simulink model "RL_Traction_motor_torch"  (R2022a)
settings: Solver=FixedStepAuto  StartTime=0.0  StopTime=0.25  FixedStep=5E-6  RelTol=1e-3
model workspace (MAT data in the model file):
  Cdc = 0.001
  Jm = 0.1234
  Ki_id = 710.3004
  Ki_iq = 1061.5
  Ki_omega = 500
  Kp_id = 0.8779
  Kp_iq = 1.0744
  Kp_omega = 20
  L0 = 0.00012184
  Ld = 0.00024368
  LdMatrix = [0.000182 0.00018 0.000178 0.000177 0.000176 0.00017475 0.0001735 0.00017247 0.00017132 0.00016571 0.00016537 0.00016571 ... (735 elements, 21x35)]
  Lq = 0.00029758
  LqMatrix = [0.000217 0.000217 0.000217 0.000217 0.000217 0.0002145 0.000212 0.0002115 0.00021022 0.0002079 0.00020461 0.0002079 ... (735 elements, 21x35)]
  PmMatrix = [0.0363 0.0363 0.0363 0.0363 0.0363 0.0363 0.0363 0.0363 0.0363 0.0363 0.0363 0.0363 ... (735 elements, 21x35)]
  Pmax = 35000
  Rs = 0.010087
  Tmax = 200
  Ts = 5e-06
  Tsc = 0.0001
  V1 = 290
  Vnom = 325
  fsw = 10000
  idVec = [-250 -225 -200 -175 -150 -125 -100 -75 -50 -25 0 25 50 75 100 125 150 175 200 225 250]
  iqVec = [-425 -400 -375 -350 -325 -300 -275 -250 -225 -200 -175 -150 -125 -100 -75 -50 -25 0 25 50 75 100 125 150 175 200 225 250 275 300 325 350 375 400 425]
  p = 8
  psim = 0.044
undefined symbols (not defined in the file or in its folder): ee_sli_rtmsupport, gcbh, idMatrix, Imax, iqMatrix, rpmVec, TqVec, VdcVec
libraries: fl_lib x19, nesl_utility x13, eeGeneralControl x9, ee_lib x7, slpidlib x5, simulink x3, eeTransforms x2, eeDqVoltageLimiter x1, eePwmGeneratorTwoLevel x1, eeResolverToDigitalConverter x1
(part 1 of 3)
settings Model: Creator=USER  LastModifiedBy=USER
settings DataIOCC: ReturnWorkspaceOutputs=off
settings ModelReferenceCC: EnableRefExpFcnMdlSchedulingChecks=off
settings RTWCC: Description=Generic Real-Time Target

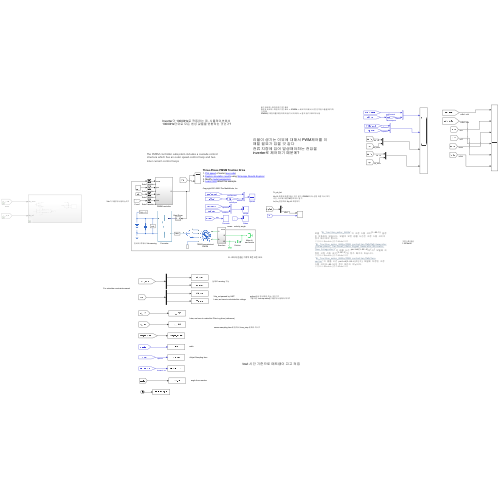
[thumbnail: Simulink's stored preview of the top-level diagram]
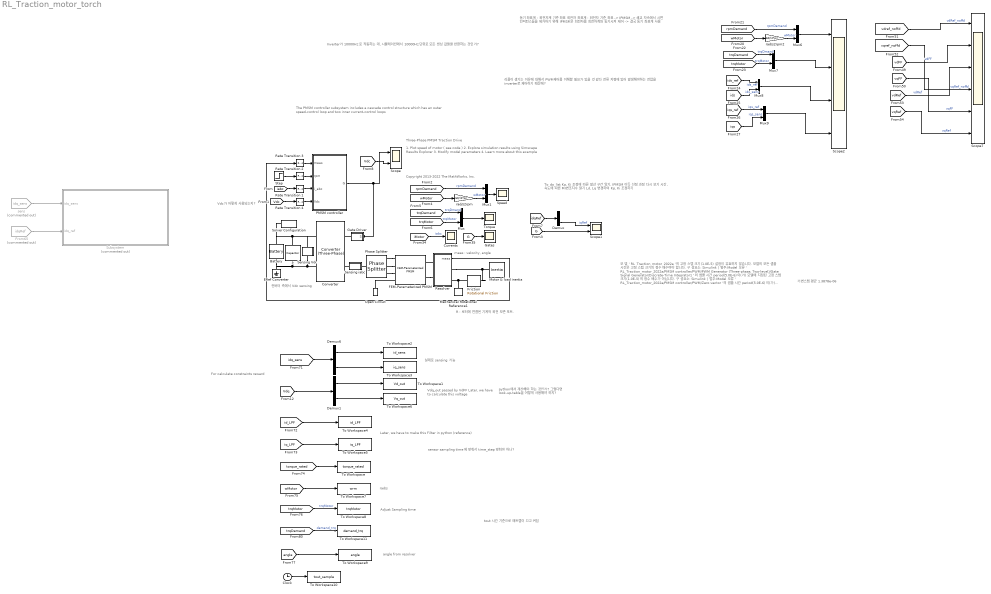
== system RL_Traction_motor_torch ==
  note: 가변스텝 평균
      | 1.3878e-06
  note: 모 델 ' RL_Traction_motor_2022a '의 고정 스텝 크기(1.0E-5) 설정이 유효하지 않습니다. 모델의 모든 샘플 시간은 고정 스텝 크기의 정수 배수여야 합니다.
      | 구 성요소: Simulink | 범주:Model 오류
      | ' RL_Traction_motor_2022a/PMSM controller/PWM/PWM Generator (Three-phase, Two-level)/Gate Signal Generator/Discrete-Time Integrator1 '의 샘플 시간 period(5.0E-6)이(가) 모델에 지정된 고정 스텝 크기(1.0E-5)의 정수 배수가 아닙니다.
      | 구 성요소: Simulink | 범주:Model 오류
      | ' RL_Traction_motor_2022a/PMSM controller/PWM/Zero vector '의 샘플 시간 period(5.0E-6)이(가) 모델에 지정된 고정 스텝 크기(1.0E-5)의 정수 배수가 아닙니다.
      | 구 성요소: Simulink | 범주:Model 오류
  note: Later, we have to make this Filter in python (reference)
  note: python에서 계산해야 하는 것인가?
      | 그렇다면 look-up-table을 어떻게 사용해야 하지?
  note: tout 시간 기준으로 매트랩이 끄고 켜짐
  note: sensor sampling time에 맞춰서 time_step 맞춰야 하나?
  note: 동기 좌표계 : 회전자계 기준 좌표
      | 회전자 좌표계 : 회전자 기준 좌표 -> IPMSM -> 쇄교 자속에서 시변 인덕턴스들을 제거하기 위해
      | IPMSM은 회전자를 회전자계와 동기시켜 제어 -> 결국 동기 좌표계 사용
  note: angle from resolver
  note: rad/s
  note: Adjust Sampling time
  note: 실제로 sensing 가능
  note: For calculate constraints reward
  note: Vdq_out passed by VdFF
      | Later, we have to calculate this voltage
  note: Inverter가 10000Hz로 작동하는 데, 시뮬레이션에서 10000Hz단위로 모든 센싱 값들을 반환하는 것인가?
  note: 리플이 생기는 이유에 대해서 PWM제어를 이해할 필요가 있을 것 같다
      | 전류 지령에 있어 발생해야하는 전압을 inverter로 제어하기 때문에?
  note: To_do_list
      |
      | Kp, Ki 조정에 따른 발산 구간 알기, IPMSM 이득 선정 과정 다시 보기
      | 시간, 속도에 따른 MI변조지수 알기
      | Ld, Lq 변경하여 Kp, Ki 조정하기
  note: Vdc가 어떻게 사용되는지?
  note: R : 로터에 연결된 기계적 회전 보존 포트.
  note: 컨버터 측에서 Vdc sensing
  note: The PMSM controller subsystem includes a cascade control structure which has an outer speed-control loop and two inner current-control loops
  note: Copyright 2013-2022 The MathWorks, Inc.
  note: meas : velocity, angle
  note: 1. Plot speed of motor ( see code )
      | 2. Explore simulation results using Simscape Results Explorer
      | 3. Modify model parameters
      | 4. Learn more about this example
  note: Three-Phase PMSM Traction Drive
  Battery : ee_lib/Sources/Battery  Vnom=Vnom V  prm_dir=ee.enum.batterybasic.prm_dir.disabled  R1_dis=2 Ohm  R1_ch=2 Ohm  R1=0.1 Ohm  prm_AH=ee.enum.batterybasic.prm_AH.infinite  AH=50 A*hr  V1=11.5 V  AH1=25 A*hr  prm_R2=ee.enum.batterybasic.prm_R2.disabled  R2=2000 Ohm  prm_dyn=ee.enum.batterybasic.prm_dyn.off  Rp1=0.005 Ohm  tau1=30 s  Rp2=0.005 Ohm  tau2=30 s  Rp3=0.005 Ohm  tau3=30 s  Rp4=0.005 Ohm  tau4=30 s  Rp5=0.005 Ohm  tau5=30 s  prm_fade=ee.enum.batterybasic.prm_fade.disabled  N_fade=100  AH_fade=45 A*hr  R1_fade=2.02 Ohm  R1_ch_fade=2.02 Ohm  V1_fade=10.35 V  prm_age=ee.enum.batterybasic.prm_age.disabled  prm_age_OCV=ee.enum.batterybasic.prm_age_OCV.OCV  OCV_age=0.9  SOC_age=60  delta_time_age_vec=[0] d  temperature_age_vec=[273] K  OCV_scaling_age=2.2134e6  OCV_offset_age=1.632e6  temp_exp_age=0.515833569 V  t_exp_age=0.75  i_specify=off  i_priority=None  i=0 A  i_nominal_specify=off  i_nominal_unit=A  i_nominal_value=1  v_specify=off  v_priority=None  v=0 V  v_nominal_specify=off  v_nominal_unit=V  v_nominal_value=1  charge_specify=on  charge_priority=High  charge=50 A*hr  charge_nominal_specify=off  charge_nominal_unit=A*hr  charge_nominal_value=1  num_cycles_specify=off  num_cycles_priority=High  num_cycles=0  num_cycles_nominal_specify=off  num_cycles_nominal_unit=1  num_cycles_nominal_value=1  Tmeas=298.15 K  Tmeas_age=298.15 K  Vnom_T2=12 V  R1_T2=2.2 Ohm  R1_T2_dis=2.2 Ohm  R1_T2_ch=2.2 Ohm  V1_T2=11.4 V  R2_T2=2200 Ohm  Rp1_T2=0.005 Ohm  tau1_T2=30 s  Rp2_T2=0.005 Ohm  tau2_T2=30 s  Rp3_T2=0.005 Ohm  tau3_T2=30 s  Rp4_T2=0.005 Ohm  tau4_T2=30 s  Rp5_T2=0.005 Ohm  tau5_T2=30 s  Tmeas2=273.15 K  thermal_mass=30000 J/K  temperature_specify=off  temperature_priority=High  temperature=298.15 K  temperature_nominal_specify=off  temperature_nominal_unit=K  temperature_nominal_value=1
  C : fl_lib/Electrical/Electrical Elements/Capacitor  c=Cdc F  r=0.01 Ohm  g=0 1/Ohm  i_specify=off  i_priority=None  i=0 A  i_nominal_specify=off  i_nominal_unit=A  i_nominal_value=1  v_specify=off  v_priority=None  v=0 V  v_nominal_specify=off  v_nominal_unit=V  v_nominal_value=1  vc_specify=on  vc_priority=None  vc=Vnom V  vc_nominal_specify=off  vc_nominal_unit=V  vc_nominal_value=1
      settings: SourceProductBaseCode=PW,SS,VE
  Clock : Clock
  Converter : ee_lib/Semiconductors & Converters/Converters/Converter (Three-Phase)  port_option=ee.enum.threePhasePort.composite  device_type=ee.enum.converters.switchingdevice.igbt  Vf=0.8 V  Ron=0.1 Ohm  Rds=0.001 Ohm  Goff=1e-5 1/Ohm  Vgt=1 V  Vgt_off=-1 V  Ih=1 A  Vth=0.5 V  diode_param=ee.enum.converters.protectiondiode.nodynamics  diode_Vf=0.8 V  diode_Ron=0.1 Ohm  diode_Goff=1e-5 1/Ohm  diode_C=50 nF  diode_iRM=-235 A  diode_iF=300 A  diode_idot=-50 A/us  diode_trr_param=ee.enum.converters.diodetrr.trr_factor  diode_trr_factor=3  diode_trr=15 us  diode_Qrr=1.5e+3 s*uA  snubber_type=ee.enum.converters.snubber.exclude  Cs=1e-7 F  Rs=0.1 Ohm
      settings: SourceProductBaseCode=PS
  Currents : Scope
  Demux : Demux  Outputs=2
  Demux1 : Demux  Outputs=2
  Demux6 : Demux  Outputs=2
  ERef Converter : fl_lib/Electrical/Electrical Elements/Electrical Reference
      settings: SourceProductBaseCode=PW,SS,VE
  FEM-Parameterized PMSM : ee_lib/Electromechanical/Permanent Magnet/FEM-Parameterized PMSM  parameterization=2  winding_type=ee.enum.statorconnection.wye  iVec=[-2, 0, 2] A  xVec=[0, 20, 40, 60] deg  dfluxdiMatrix=0.0002 * ones(3, 4) Wb/A  dfluxdxMatrix=[0, -.16, .16, 0; 0, -.16, .16, 0; 0, -.16, .16, 0] Wb/rad  calculate_torque_matrix=1  TorqueMatrix=zeros(3, 3, 3, 4) N*m  idVec1=idVec A  iqVec1=iqVec A  LdMatrix=LdMatrix H  LqMatrix=LqMatrix H  PmMatrix=PmMatrix Wb  N=p  interp_method=simscape.enum.interpolation.smooth  Rs=Rs Ohm  Ms=0.00002 H  L0=0.00016 H  loss_param=ee.enum.fem_motor.ironLossesExtended.empirical  losses_oc=[500 1500 0] W  losses_sc=[200 600 0] W  f_losses=220 Hz  Isc_losses=450 A  Inertia=0 kg*m^2  lam=0 N*m/(rad/s)  i_d_specify=off  i_d_priority=None  i_d=0 A  i_d_nominal_specify=off  i_d_nominal_unit=A  i_d_nominal_value=1  i_q_specify=off  i_q_priority=None  i_q=0 A  i_q_nominal_specify=off  i_q_nominal_unit=A  i_q_nominal_value=1  torque_specify=off  torque_priority=None  torque=0 N*m  torque_nominal_specify=off  torque_nominal_unit=N*m  torque_nominal_value=1  angular_velocity_specify=on  angular_velocity_priority=None  angular_velocity=0 rpm  angular_velocity_nominal_specify=off  angular_velocity_nominal_unit=rpm  angular_velocity_nominal_value=1  angular_position_specify=on  angular_position_priority=High  angular_position=-pi/2/p rad  angular_position_nominal_specify=off  angular_position_nominal_unit=deg  angular_position_nominal_value=1  Tmeas=298.15 K  alpha=3.93e-3 1/K  alpha_flux=-0.001 1/K  stator_thermal_mass=100 J/K  stator_initial_temperatures=[298.15, 298.15, 298.15] K  rotor_thermal_mass=200 J/K  rotor_initial_temperature=298.15 K  Rm_percent_rotor=90  Rd_percent_rotor=30  idVec=[-200, 0, 200] A  iqVec=[-200, 0, 200] A  dfluxAdiaMatrix3D=zeros(3, 3, 4) Wb/A  dfluxAdibMatrix3D=zeros(3, 3, 4) Wb/A  dfluxAdicMatrix3D=zeros(3, 3, 4) Wb/A  dfluxAdxMatrix3D=zeros(3, 3, 4) Wb/rad  TorqueMatrix3D=zeros(3, 3, 4) N*m  iaVec=[-200, 0, 200] A  ibVec=[-200, 0, 200] A  icVec=[-200, 0, 200] A  dfluxAdiaMatrix=zeros(3, 3, 3, 4) Wb/A  dfluxAdibMatrix=zeros(3, 3, 3, 4) Wb/A  dfluxAdicMatrix=zeros(3, 3, 3, 4) Wb/A  dfluxAdxMatrix=zeros(3, 3, 3, 4) Wb/rad  param_dq0=ee.enum.fem_motor.fluxTabulationOption.DQcartesian  winding_type_dq0=ee.enum.statorconnection.wye  expose_neutral_port=ee.enum.fem_motor.exposeNeutralPort.no  nPolePairs=4  parks_type=ee.enum.fem_motor.parksType.QleadsD_AphaseToDaxis  idVec2=[-200, 0, 200] A  iqVec2=[-200, 0, 200] A  magVec2=[0, 100, 200] A  betaVec2=[-180, -90, 0, 90, 180] deg  xVec2=[0, 5, 10, 15, 20, 25, 30] deg  fluxD_dq0=zeros(3, 3, 7) Wb  fluxQ_dq0=zeros(3, 3, 7) Wb  fluxA_dq0=zeros(3, 3, 7) Wb  Torque_dq0=ones(3, 3, 7) N*m  fluxD_IBX=zeros(3, 5, 7) Wb  fluxQ_IBX=zeros(3, 5, 7) Wb  fluxA_IBX=zeros(3, 5, 7) Wb  Torque_IBX=zeros(3, 5, 7) N*m  rotorLossCoeff_k_h_DQ=zeros(3, 3) W/Hz  rotorLossCoeff_k_J_DQ=zeros(3, 3) W/Hz^2  rotorLossCoeff_k_ex_DQ=zeros(3, 3) W/Hz^(3/2)  rotorLossCoeff_k_h_IB=zeros(3, 5) W/Hz  rotorLossCoeff_k_J_IB=zeros(3, 5) W/Hz^2  rotorLossCoeff_k_ex_IB=zeros(3, 5) W/Hz^(3/2)  statorLossCoeff_k_h_DQ=zeros(3, 3) W/Hz  statorLossCoeff_k_J_DQ=zeros(3, 3) W/Hz^2  statorLossCoeff_k_ex_DQ=zeros(3, 3) W/Hz^(3/2)  statorLossCoeff_k_h_IB=zeros(3, 5) W/Hz  statorLossCoeff_k_J_IB=zeros(3, 5) W/Hz^2  statorLossCoeff_k_ex_IB=zeros(3, 5) W/Hz^(3/2)  wVec=[1000, 2000] rpm  rotorLossTable_DQ=zeros(3, 3, 2) W  rotorLossTable_IB=zeros(3, 5, 2) W  statorLossTable_DQ=zeros(3, 3, 2) W  statorLossTable_IB=zeros(3, 5, 2) W  electrical_torque_before_iron_losses_specify=off  electrical_torque_before_iron_losses_priority=None  electrical_torque_before_iron_losses=0 N*m  electrical_torque_before_iron_losses_nominal_specify=off  electrical_torque_before_iron_losses_nominal_unit=N*m  electrical_torque_before_iron_losses_nominal_value=1  Qrotor_specify=off  Qrotor_priority=None  Qrotor=0 J/s  Qrotor_nominal_specify=off  Qrotor_nominal_unit=J/s  Qrotor_nominal_value=1  Qstator_specify=off  Qstator_priority=None  Qstator=0 J/s  Qstator_nominal_specify=off  Qstator_nominal_unit=J/s  Qstator_nominal_value=1
      settings: SourceProductBaseCode=PS  LogSimulationData=on  InternalSimscapePortConfiguration="{\"Bottom\":[],\"Left\":[{\"id\":\"a\",\"label\":\"a\",\"type\":\"foundation.electrical.electrical\"},{\"id\":\"b\",\"label\":\"b\",\"type\":\"foundation.electrical.electrical\"},{\"id\":\"c\",\"label\":\"c\",\"type\":\"foundation.electrical.electrical\"},{\"id\":\"n\",\"label\":\"n\",\"type\":\"foundation.electrical.electrical\"}],\"Right\":[{\"id\":\"R\",\"label\":\"R\",\"type\":\"foundation.mechanical.rotational.rotational\"},{\"id\":\"C\",\"label\":\"C\",\"type\":\"foundation.mechanical.rotational.rotational\"}],\"Top\":[]}"
  Friction : fl_lib/Mechanical/Rotational Elements/Rotational Friction  brkwy_trq=25 N*m  brkwy_vel=0.1 rad/s  Col_trq=20 N*m  visc_coef=0.1 N*m/(rad/s)  w_specify=off  w_priority=None  w=0 rad/s  w_nominal_specify=off  w_nominal_unit=rad/s  w_nominal_value=1  t_specify=off  t_priority=None  t=0 N*m  t_nominal_specify=off  t_nominal_unit=N*m  t_nominal_value=1
      settings: SourceProductBaseCode=PW,SS,VE
  From65 : From  Commented=on  GotoTag=idqRef  TagVisibility=global
  Gate Driver : Subsystem
  Gates : Scope
  Mechanical Rotational Reference1 : fl_lib/Mechanical/Rotational Elements/Mechanical Rotational Reference
      settings: SourceProductBaseCode=PW,SS,VE
  Motor & load inertia : fl_lib/Mechanical/Rotational Elements/Inertia  inertia=Jm kg*m^2  num_ports=foundation.enum.numPorts2.one  w_specify=on  w_priority=High  w=0 rpm  w_nominal_specify=off  w_nominal_unit=rad/s  w_nominal_value=1  t_specify=off  t_priority=High  t=0 N*m  t_nominal_specify=off  t_nominal_unit=N*m  t_nominal_value=1
      settings: SourceProductBaseCode=PW,SS,VE
  Mux{,1,6..9} (6 alike) : Mux  Inputs=2
  Open Circuit : fl_lib/Electrical/Electrical Elements/Open Circuit  v_specify=off  v_priority=None  v=0 V  v_nominal_specify=off  v_nominal_unit=V  v_nominal_value=1
      settings: SourceProductBaseCode=PW,SS,VE
  PMSM controller : Subsystem
  Phase Splitter : ee_lib/Connectors & References/Phase Splitter
      settings: SourceProductBaseCode=PS
  Rate Transition {1..4} (4 alike) : RateTransition  OutPortSampleTime=Tsc
  Resolver : Subsystem
  Scope : Scope  NumInputPorts=2
  Scope1 : Scope  NumInputPorts=2
  Scope2 : Scope  NumInputPorts=4
  Scope7 : Scope  NumInputPorts=6
  Sensing Vdc : Subsystem
      mask Display: disp('vdc')
  Sensing iabc : Subsystem
      mask Display: disp('iabc')
  Solver Configuration : nesl_utility/Solver Configuration  PhysicalDomain=network_engine_domain  SubClassName=solver  LeftPortType=input  RightPortType=generic  Tones=[]  Harmonics=[]  SimulateNoise=off  Profile=off  UseLocalSampling=off  EnableSwitchedLinearOptims=on  FrequencyDomain=off  UseCCode=off  RelTol=0.001  AbsTol=1e-06  MinStep=1e-09  ToWorkspace=off  RevertToSquareIcSolve=off  NumHomotopyIterations=100  PhasorMode=off  PhasorModeNumHarmonics=1  IndexReductionMethod=DerivativeReplacement  DoDC=off  ResidualTolerance=1e-9  UseLocalSolver=off  LocalSolverChoice=NE_BACKWARD_EULER_ADVANCER  LocalSolverSampleTime=Ts  DoFixedCost=on  MaxNonlinIter=4  MaxModeIter=2  ComputeImpulses=off  ImpulseIterations=2  LinearAlgebra=auto  LinearAlgebraNumThread=0  EquationFormulation=NE_TIME_EF  DelaysMemoryBudget=1024  AutomaticFiltering=on  FilteringTimeConstant=0.001  PartitionStorageMethod=AS_NEEDED  PartitionMemoryBudget=1024  PartitionMethod=FAST
      settings: SourceProductBaseCode=SS,PW,VE
  Speed : Scope
  Step : Step  Time=0.001  After=1000  SampleTime=0
  Subsystem : Subsystem  Commented=on
  To Workspace : ToWorkspace  VariableName=torque_rated  SampleTime=-1
      settings: MaxDataPoints=1  Save2DSignal=2-D array (concatenate along first dimension)
  To Workspace1 : ToWorkspace  VariableName=Vd_out  SampleTime=-1
      settings: MaxDataPoints=1  Save2DSignal=2-D array (concatenate along first dimension)
  To Workspace10 : ToWorkspace  VariableName=tout_sample  SampleTime=Tsc
      settings: MaxDataPoints=1  Save2DSignal=2-D array (concatenate along first dimension)
  To Workspace11 : ToWorkspace  VariableName=demand_trq  SampleTime=Tsc
      settings: MaxDataPoints=1  Save2DSignal=2-D array (concatenate along first dimension)
  To Workspace2 : ToWorkspace  VariableName=id_sens  SampleTime=-1
      settings: MaxDataPoints=1  Save2DSignal=2-D array (concatenate along first dimension)
  To Workspace3 : ToWorkspace  VariableName=iq_sens  SampleTime=-1
      settings: MaxDataPoints=1  Save2DSignal=2-D array (concatenate along first dimension)
  To Workspace4 : ToWorkspace  VariableName=id_LPF  SampleTime=-1
      settings: MaxDataPoints=1  Save2DSignal=2-D array (concatenate along first dimension)
  To Workspace5 : ToWorkspace  VariableName=iq_LPF  SampleTime=-1
      settings: MaxDataPoints=1  Save2DSignal=2-D array (concatenate along first dimension)
  To Workspace6 : ToWorkspace  VariableName=Vq_out  SampleTime=-1
      settings: MaxDataPoints=1  Save2DSignal=2-D array (concatenate along first dimension)
  To Workspace7 : ToWorkspace  VariableName=wrm  SampleTime=-1
      settings: MaxDataPoints=1  Save2DSignal=2-D array (concatenate along first dimension)
  To Workspace8 : ToWorkspace  VariableName=trqMotor  SampleTime=Tsc
      settings: MaxDataPoints=1  Save2DSignal=2-D array (concatenate along first dimension)
  To Workspace9 : ToWorkspace  VariableName=angle  SampleTime=Tsc
      settings: MaxDataPoints=1  Save2DSignal=2-D array (concatenate along first dimension)
  Torque : Scope
  rad/s2rpm : Gain  Gain=60/(2*pi)
  rad/s2rpm2 : Gain  Gain=60/(2*pi)
  sens : From  Commented=on  GotoTag=idq_sens  TagVisibility=global
  wires:
  Rate Transition 3/1 -> PMSM controller/1(meas)
  [iabc] -> Rate Transition 1/1
  Mux1/1 -> Speed/1
  [iMotor] -> Currents/1  "iabc"
  Rate Transition 1/1 -> PMSM controller/3(i_abc)
  [trqDemand] -> Mux/1  "trqDmand"
  Resolver/1(meas) -> Rate Transition 3/1
  Mux/1 -> Torque/1
  [wMotor] -> rad/s2rpm/1
  PMSM controller/1(G) -> Scope/1, Gate Driver/1(S)
  rad/s2rpm/1 -> Mux1/2  "wMotor"
  [Vdc] -> Rate Transition 4/1
  Step/1 -> Rate Transition 2/1
  [G] -> Gates/1
  [trqMotor] -> Mux/2  "trqMotor"
  Rate Transition 4/1 -> PMSM controller/4(Vdc)
  Rate Transition 2/1 -> PMSM controller/2(rpm)
  [rpmDemand] -> Mux1/1  "rpmDemand"
  [G] -> Scope1/2
  [idqRef] -> Demux/1
  Demux/2 -> Scope1/1  "iqRef"
  [Vdc] -> Scope/2
  Mux6/1 -> Scope2/1
  [wMotor] -> rad/s2rpm2/1
  rad/s2rpm2/1 -> Mux6/2  "wMotor"
  [rpmDemand] -> Mux6/1  "rpmDemand"
  [trqDemand] -> Mux7/1  "trqDmand"
  [trqMotor] -> Mux7/2  "trqMotor"
  Mux7/1 -> Scope2/2
  [ids_ref] -> Mux8/1  "ids_ref"
  [ids] -> Mux8/2  "ids_sens"
  Mux8/1 -> Scope2/3
  [iqs] -> Mux9/2  "iqs_sens"
  [iqs_ref] -> Mux9/1  "iqs_ref"
  Mux9/1 -> Scope2/4
  [vqFF] -> Scope7/5  "vqFF"
  [vdRef] -> Scope7/3  "vdRef"
  [vqref_noffd] -> Scope7/4  "vqRef_noffd"
  [vdFF] -> Scope7/2  "vdFF"
  [vqRef] -> Scope7/6  "vqRef"
  [vdref_noffd] -> Scope7/1  "vdRef_noffd"
  sens/1 -> Subsystem/1(idq_sens)
  From65/1 -> Subsystem/2(idq_ref)
  Demux6/2 -> To Workspace3/1
  [idq_sens] -> Demux6/1
  Demux6/1 -> To Workspace2/1
  [iq_LPF] -> To Workspace5/1
  [id_LPF] -> To Workspace4/1
  [torque_rated] -> To Workspace/1
  Demux1/1 -> To Workspace1/1
  Demux1/2 -> To Workspace6/1
  [Vdq] -> Demux1/1
  [wMotor] -> To Workspace7/1
  [trqMotor] -> To Workspace8/1  "trqMotor"
  [angle] -> To Workspace9/1
  Clock/1 -> To Workspace10/1
  [trqDemand] -> To Workspace11/1  "demand_trq"
  connections:
  C/RConn1 -- Battery/RConn1 -- ERef Converter/LConn1 -- Sensing Vdc/RConn1 -- Converter/RConn2
  Sensing Vdc/LConn1 -- Converter/RConn1 -- Solver Configuration/RConn1 -- Battery/LConn1 -- C/LConn1
  Friction/LConn1 -- Motor & load inertia/LConn1 -- Resolver/RConn1
  Friction/RConn1 -- Mechanical Rotational Reference1/LConn1 -- Resolver/RConn2
  FEM-Parameterized PMSM/RConn2 -- Resolver/LConn2
  Phase Splitter/RConn1 -- FEM-Parameterized PMSM/LConn1
  Open Circuit/LConn1 -- FEM-Parameterized PMSM/LConn4
  Phase Splitter/RConn2 -- FEM-Parameterized PMSM/LConn2
  Gate Driver/RConn1 -- Converter/LConn1
  Phase Splitter/RConn3 -- FEM-Parameterized PMSM/LConn3
  Phase Splitter/LConn1 -- Sensing iabc/RConn1
  Sensing iabc/LConn1 -- Converter/LConn2
  Resolver/LConn1 -- FEM-Parameterized PMSM/RConn1

== system RL_Traction_motor_torch/Gate Driver ==
  S : Inport
  Demux : Demux  Outputs=6
  Scope : Scope  NumInputPorts=6
  Simulink-PS Converter{1..6} (6 alike) : nesl_utility/Simulink-PS Converter  PhysicalDomain=network_engine_domain  SubClassName=ps_input  LeftPortType=input  RightPortType=output  PseudoPeriodic=off  Frequencies=[]  NoiseDistribution=none  NoiseParameters=[]  Unit=1  AffineConversion=off  FilteringAndDerivatives=zero  SimscapeFilterOrder=1  InputFilterTimeConstant=0.001  UdotUserProvided=1
      settings: SourceProductBaseCode=SS,PW,VE
  Six-Pulse Gate Multiplexer : ee_lib/Semiconductors & Converters/Converters/Six-Pulse Gate Multiplexer  port_option=ee.enum.controlport.ps
      settings: SourceProductBaseCode=PS
  G : PMIOPort  Side=Right
  wires:
  Demux/1 -> Simulink-PS Converter1/1, Scope/1
  Demux/4 -> Simulink-PS Converter4/1, Scope/4
  Demux/2 -> Simulink-PS Converter2/1, Scope/2
  Demux/3 -> Scope/3, Simulink-PS Converter3/1
  Demux/5 -> Scope/5, Simulink-PS Converter5/1
  Demux/6 -> Scope/6, Simulink-PS Converter6/1
  S/1 -> Demux/1
  connections:
  G/RConn1 -- Six-Pulse Gate Multiplexer/RConn1
  Simulink-PS Converter5/RConn1 -- Six-Pulse Gate Multiplexer/LConn5
  Simulink-PS Converter4/RConn1 -- Six-Pulse Gate Multiplexer/LConn4
  Simulink-PS Converter6/RConn1 -- Six-Pulse Gate Multiplexer/LConn6
  Simulink-PS Converter3/RConn1 -- Six-Pulse Gate Multiplexer/LConn3
  Simulink-PS Converter2/RConn1 -- Six-Pulse Gate Multiplexer/LConn2
  Simulink-PS Converter1/RConn1 -- Six-Pulse Gate Multiplexer/LConn1

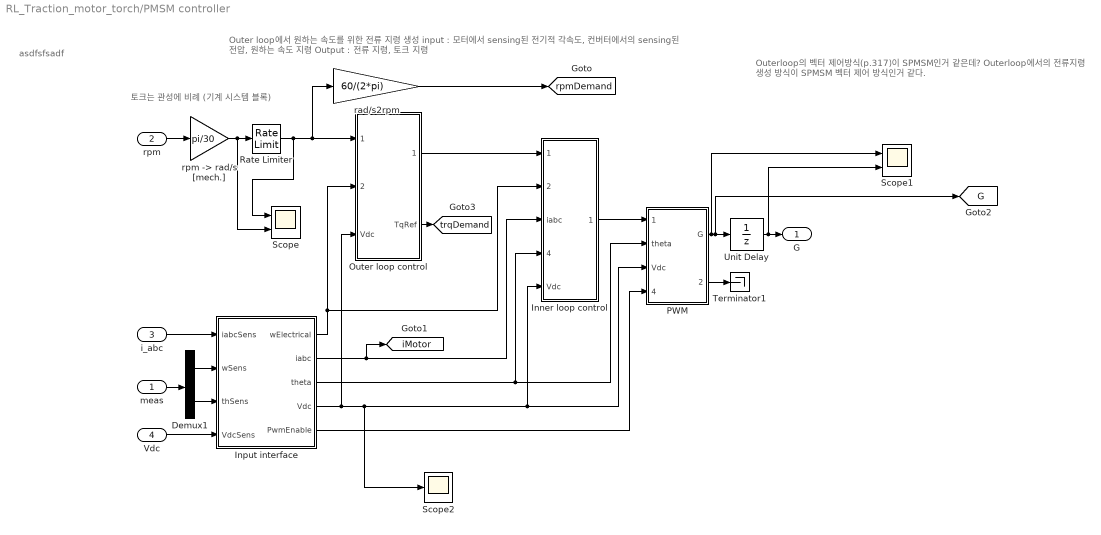
== system RL_Traction_motor_torch/PMSM controller ==
  note: asdfsfsadf
  note: Outerloop의 벡터 제어방식(p.317)이 SPMSM인거 같은데?
      | Outerloop에서의 전류지령 생성 방식이 SPMSM 벡터 제어 방식인거 같다.
  note: Outer loop에서 원하는 속도를 위한 전류 지령 생성
      | input : 모터에서 sensing된 전기적 각속도, 컨버터에서의 sensing된 전압, 원하는 속도 지령
      | Output : 전류 지령, 토크 지령
  note: 토크는 관성에 비례 (기계 시스템 블록)
  meas : Inport
  rpm : Inport  Port=2
  i_abc : Inport  Port=3
  Vdc : Inport  Port=4
  Demux1 : Demux  Outputs=2
  Inner loop control : Subsystem
  Input interface : Subsystem
  Outer loop control : Subsystem
  PWM : Subsystem
  Rate Limiter : RateLimiter  RisingSlewLimit=Tmax/Jm  FallingSlewLimit=-Tmax/Jm  SampleTimeMode=inherited
  Scope : Scope  NumInputPorts=2
  Scope1 : Scope  NumInputPorts=2
  Scope2 : Scope
  Terminator1 : Terminator
  Unit Delay : UnitDelay  SampleTime=Ts  HasFrameUpgradeWarning=on
  rad/s2rpm : Gain  Gain=60/(2*pi)
  "rpm -> rad/s [mech.]" : Gain  Gain=pi/30
  G : Outport  VectorParamsAs1DForOutWhenUnconnected=off
  tag scope: G=global, iMotor=global, rpmDemand=global, trqDemand=global
  wires:
  meas/1 -> Demux1/1
  Demux1/1 -> Input interface/2(wSens)
  rpm/1 -> "rpm -> rad/s [mech.]"/1
  "rpm -> rad/s [mech.]"/1 -> Scope/2, Rate Limiter/1
  PWM/1(G) -> Scope1/1, [G], Unit Delay/1
  Input interface/1(wElectrical) -> Outer loop control/2(wElectrical), Inner loop control/2(wElectrical)
  Vdc/1 -> Input interface/4(VdcSens)
  Outer loop control/1(idqRef) -> Inner loop control/1(idq_ref)
  Rate Limiter/1 -> Scope/1, Outer loop control/1(Reference), rad/s2rpm/1
  Input interface/4(Vdc) -> Scope2/1, PWM/3(Vdc), Inner loop control/5(Vdc), Outer loop control/3(Vdc)
  Input interface/5(PwmEnable) -> PWM/4(PwmEnable)
  Input interface/3(theta) -> PWM/2(theta), Inner loop control/4(theta)
  Inner loop control/1(vdqRef) -> PWM/1(vdqRef)
  Outer loop control/2(TqRef) -> [trqDemand]
  Input interface/2(iabc) -> Inner loop control/3(iabc), [iMotor]
  Demux1/2 -> Input interface/3(thSens)
  i_abc/1 -> Input interface/1(iabcSens)
  PWM/2(ModWave) -> Terminator1/1
  rad/s2rpm/1 -> [rpmDemand]
  Unit Delay/1 -> Scope1/2, G/1

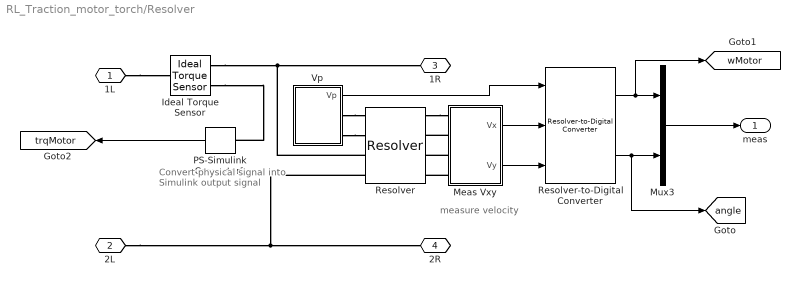
== system RL_Traction_motor_torch/Resolver ==
  note: measure velocity
  note: Convert physical signal into Simulink output signal
  Ideal Torque Sensor : fl_lib/Mechanical/Mechanical Sensors/Ideal Torque Sensor
      settings: SourceProductBaseCode=PW,SS,VE
  Meas Vxy : Subsystem
  Mux3 : Mux  Inputs=2
  PS-Simulink Converter2 : nesl_utility/PS-Simulink Converter  PhysicalDomain=network_engine_domain  SubClassName=ps_output  LeftPortType=input  RightPortType=output  PseudoPeriodic=off  Frequencies=[]  VectorFormat=1-D array  Unit=N*m  AffineConversion=off
      settings: SourceProductBaseCode=SS,PW,VE
  Resolver : ee_lib/Sensors & Transducers/Resolver  parameterization=1  ratio=0.5  Rr=70 Ohm  Rs=180 Ohm  Xr=100 Ohm  Xs=300 Ohm  omega=10 kHz  Lr=0.0016 H  Ls=0.0048 H  k=0.35  N=4  theta_specify=off  theta_priority=High  theta=0 deg  theta_nominal_specify=off  theta_nominal_unit=deg  theta_nominal_value=1
      settings: SourceProductBaseCode=PS  InternalSimscapePortConfiguration="{\"Bottom\":[],\"Left\":[{\"id\":\"p1\",\"label\":\"p1\",\"type\":\"foundation.electrical.electrical\"},{\"id\":\"p2\",\"label\":\"p2\",\"type\":\"foundation.electrical.electrical\"},{\"id\":\"R\",\"label\":\"R\",\"type\":\"foundation.mechanical.rotational.rotational\"},{\"id\":\"C\",\"label\":\"C\",\"type\":\"foundation.mechanical.rotational.rotational\"}],\"Right\":[{\"id\":\"x1\",\"label\":\"x1\",\"type\":\"foundation.electrical.electrical\"},{\"id\":\"x2\",\"label\":\"x2\",\"type\":\"foundation.electrical.electrical\"},{\"id\":\"y1\",\"label\":\"y1\",\"type\":\"foundation.electrical.electrical\"},{\"id\":\"y2\",\"label\":\"y2\",\"type\":\"foundation.electrical.electrical\"}],\"Top\":[]}"
  Resolver-to-Digital Converter : eeResolverToDigitalConverter/Resolver-to-Digital Converter  N=4  Kp=15  Ki=2.5e5  theta0=0  Ts=Ts
      settings: SourceProductBaseCode=PS
  Vp : Subsystem
  1L : PMIOPort  Side=Left
  2L : PMIOPort  Port=2  Side=Left
  1R : PMIOPort  Port=3  Side=Right
  2R : PMIOPort  Port=4  Side=Right
  meas : Outport  VectorParamsAs1DForOutWhenUnconnected=off
  tag scope: angle=global, trqMotor=global, wMotor=global
  wires:
  PS-Simulink Converter2/1 -> [trqMotor]
  Mux3/1 -> meas/1
  Meas Vxy/1(Vx) -> Resolver-to-Digital Converter/2
  Vp/1(Vp) -> Resolver-to-Digital Converter/1
  Resolver-to-Digital Converter/1 -> [wMotor], Mux3/1
  Resolver-to-Digital Converter/2 -> [angle], Mux3/2
  Meas Vxy/2(Vy) -> Resolver-to-Digital Converter/3
  connections:
  Ideal Torque Sensor/RConn2 -- PS-Simulink Converter2/LConn1
  1L/RConn1 -- Ideal Torque Sensor/LConn1
  2L/RConn1 -- Resolver/LConn4 -- 2R/RConn1
  Ideal Torque Sensor/RConn1 -- Resolver/LConn3 -- 1R/RConn1
  Meas Vxy/LConn2 -- Resolver/RConn2
  Resolver/RConn1 -- Meas Vxy/LConn1
  Meas Vxy/LConn3 -- Resolver/RConn3
  Meas Vxy/LConn4 -- Resolver/RConn4
  Vp/RConn1 -- Resolver/LConn1
  Vp/RConn2 -- Resolver/LConn2
